simulink model "Task1new"  (R2022a)
settings: Solver=FixedStepAuto  StartTime=0.0  StopTime=20  FixedStep=0.0001  RelTol=1e-3
undefined symbols (not defined in the file): a1, a2, a3, k1, k2
libraries: simulink_extras x1
settings Model: Creator=Family  LastModifiedBy=Family

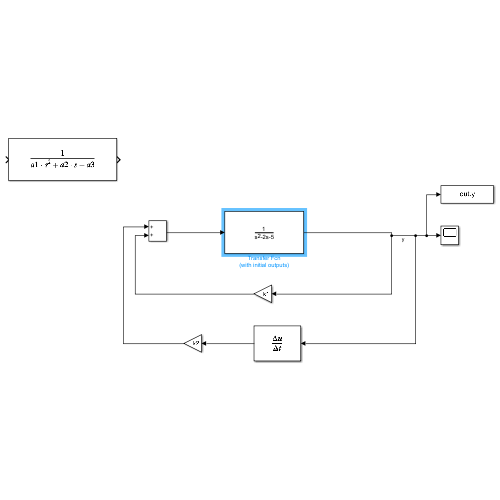
[thumbnail: Simulink's stored preview of the top-level diagram]
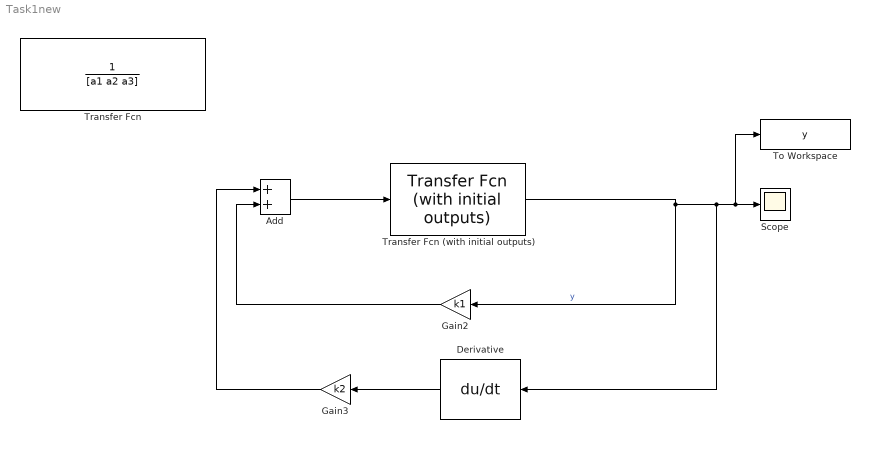
== system Task1new ==
  Add : Sum
  Derivative : Derivative
  Gain2 : Gain  Gain=k1
  Gain3 : Gain  Gain=k2
  Scope : Scope
  To Workspace : ToWorkspace  VariableName=y  SaveFormat=Timeseries  SampleTime=-1
  Transfer Fcn : TransferFcn  Denominator=[a1 a2 a3]
  Transfer Fcn (with initial outputs) : simulink_extras/Additional Linear/Transfer Fcn (with initial outputs)  N=[1]  D=[a1 a2 a3]  Y0=.5  U0=20
  wires:
  Transfer Fcn (with initial outputs)/1 -> Gain2/1, Derivative/1, To Workspace/1, Scope/1  "y"
  Derivative/1 -> Gain3/1
  Gain2/1 -> Add/2
  Gain3/1 -> Add/1
  Add/1 -> Transfer Fcn (with initial outputs)/1
